simulink model "implementationballandbeam"  (R2015a)
settings: Solver=ode1  StartTime=0.0  StopTime=25  FixedStep=0.002  RelTol=1e-3
libraries: simulink x2, simulink_extras x1
settings Model: ExtModeTrigDuration=5000  Creator=yejingzhou  LastModifiedBy=yejingzhou
settings SolverCC: PositivePriorityOrder=on
settings OptimizationCC: ExpressionDepthLimit=2147483647
settings DebuggingCC: UnderspecifiedInitializationDetection=Classic  MergeDetectMultiDrivingBlocksExec=none  SolverPrmCheckMsg=warning  StateNameClashWarn=warning
settings RTWCC: SystemTargetFile=quarc_win64.tlc  TemplateMakefile=quarc_default_tmf  Description=QUARC Win64 Target
settings STFCustomTargetCC: TargetLibSuffix=.lib  TargetPreCompLibLocation=C:\PROGRA~3\QUARC\lib\2012b\win64\release  GenerateSampleERTMain=off  GeneratePreprocessorConditionals=Disable all  CombineOutputUpdateFcns=on  ERTCustomFileBanners=off  SupportNonInlinedSFcns=on  SupportVariableSizeSignals=off  MATLABClassNameForMDSCustomization=Simulink.SoftwareTarget.GRTCustomization  CPPClassGenCompliant=on  SystemTargetFile=quarc_win64.tlc
settings GRTTargetCC: TargetPreCompLibLocation=C:\PROGRA~3\QUARC\lib\2012b\win64\release  ParMdlRefBuildCompliant=off  CompOptLevelCompliant=off  ConcurrentExecutionCompliant=off  MatFileLogging=off  ExtMode=on  ExtModeMexFile=quarc_comm

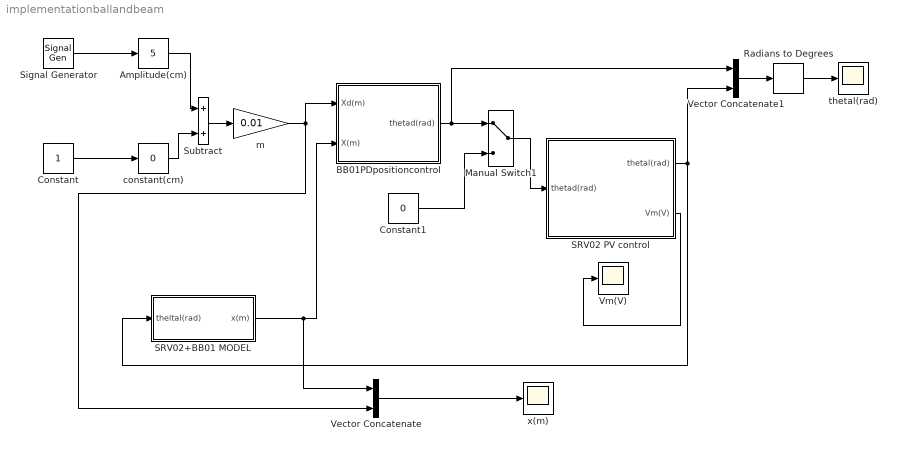
== system implementationballandbeam ==
  Amplitude(cm) : simulink/Math Operations/Slider Gain  low=-1  gain=5  high=10
  BB01PDpositioncontrol : Subsystem
  Constant : Constant
  Constant1 : Constant  Value=0
  Manual Switch1 : ManualSwitch
  Radians to Degrees : simulink_extras/Transformations/Radians to Degrees
  SRV02 PV control : Subsystem
  SRV02+BB01 MODEL : Subsystem
  Signal Generator : SignalGenerator  WaveForm=square  Frequency=0.2  Units=rad/sec
  Subtract : Sum
  Vector Concatenate : Concatenate
  Vector Concatenate1 : Concatenate
  "Vm(V) " : Scope
      settings: SaveName=ScopeData2
  constant(cm) : simulink/Math Operations/Slider Gain  low=0  gain=0  high=5
  "m " : Gain  Gain=0.01
  thetal(rad) : Scope
      settings: TimeRange=25  YMin=-125  YMax=125
  x(m) : Scope
      settings: YMin=-0.09  YMax=0.14
  wires:
  Amplitude(cm)/1 -> Subtract/1
  constant(cm)/1 -> Subtract/2
  Signal Generator/1 -> Amplitude(cm)/1
  Constant/1 -> constant(cm)/1
  Vector Concatenate/1 -> x(m)/1
  Radians to Degrees/1 -> thetal(rad)/1
  BB01PDpositioncontrol/1(thetad(rad)) -> Vector Concatenate1/1, Manual Switch1/1
  Constant1/1 -> Manual Switch1/2
  Manual Switch1/1 -> SRV02 PV control/1(thetad(rad))
  Vector Concatenate1/1 -> Radians to Degrees/1
  SRV02 PV control/1(thetal(rad)) -> SRV02+BB01 MODEL/1(theltal(rad)), Vector Concatenate1/2
  SRV02 PV control/2("Vm(V) ") -> "Vm(V) "/1
  SRV02+BB01 MODEL/1(x(m)) -> Vector Concatenate/1, BB01PDpositioncontrol/2(X(m))
  Subtract/1 -> "m "/1
  "m "/1 -> BB01PDpositioncontrol/1(Xd(m)), Vector Concatenate/2

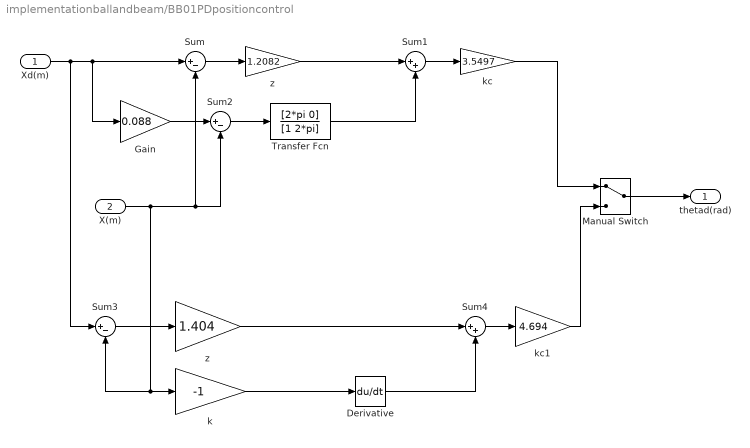
== system implementationballandbeam/BB01PDpositioncontrol ==
  Xd(m) : Inport
  X(m) : Inport  Port=2
  Derivative : Derivative
  Gain : Gain  Gain=0.088
  Manual Switch : ManualSwitch
  Sum : Sum  Inputs=|+-
  Sum1 : Sum  Inputs=|++
  Sum2 : Sum  Inputs=|+-
  Sum3 : Sum  Inputs=|+-
  Sum4 : Sum  Inputs=|++
  Transfer Fcn : TransferFcn  Numerator=[2*pi 0]  Denominator=[1 2*pi]
  k : Gain  Gain=-1
  kc : Gain  Gain=3.5497
  kc1 : Gain  Gain=4.694
  z : Gain  Gain=1.404
  "z " : Gain  Gain=1.2082
  thetad(rad) : Outport
  wires:
  Xd(m)/1 -> Sum/1, Gain/1, Sum3/1
  Sum/1 -> "z "/1
  X(m)/1 -> Sum3/2, k/1, Sum2/2, Sum/2
  "z "/1 -> Sum1/1
  Transfer Fcn/1 -> Sum1/2
  Sum1/1 -> kc/1
  Gain/1 -> Sum2/1
  Sum2/1 -> Transfer Fcn/1
  Sum3/1 -> z/1
  Sum4/1 -> kc1/1
  z/1 -> Sum4/1
  k/1 -> Derivative/1
  Derivative/1 -> Sum4/2
  Manual Switch/1 -> thetad(rad)/1
  kc1/1 -> Manual Switch/2
  kc/1 -> Manual Switch/1

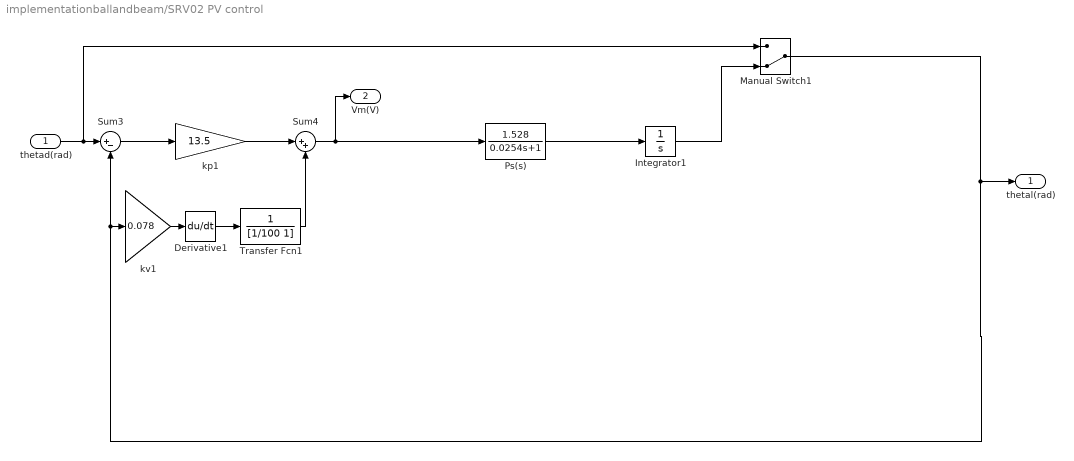
== system implementationballandbeam/SRV02 PV control ==
  thetad(rad) : Inport
  Derivative1 : Derivative
  Integrator1 : Integrator
  Manual Switch1 : ManualSwitch  CurrentSetting=0
  Ps(s) : TransferFcn  Numerator=[1.528]  Denominator=[0.0254 1]
  Sum3 : Sum  Inputs=|+-
  Sum4 : Sum  Inputs=|++
  Transfer Fcn1 : TransferFcn  Denominator=[1/100 1]
  kp1 : Gain  Gain=13.5
  kv1 : Gain  Gain=0.078
  thetal(rad) : Outport
  "Vm(V) " : Outport  Port=2
  wires:
  thetad(rad)/1 -> Manual Switch1/1, Sum3/1
  Sum3/1 -> kp1/1
  kp1/1 -> Sum4/1
  kv1/1 -> Derivative1/1
  Derivative1/1 -> Transfer Fcn1/1
  Transfer Fcn1/1 -> Sum4/2
  Ps(s)/1 -> Integrator1/1
  Manual Switch1/1 -> Sum3/2, kv1/1, thetal(rad)/1
  Sum4/1 -> Ps(s)/1, "Vm(V) "/1
  Integrator1/1 -> Manual Switch1/2

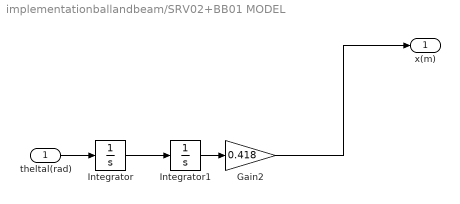
== system implementationballandbeam/SRV02+BB01 MODEL ==
  theltal(rad) : Inport
  Gain2 : Gain  Gain=0.418
  Integrator : Integrator
  Integrator1 : Integrator
  x(m) : Outport
  wires:
  Integrator/1 -> Integrator1/1
  theltal(rad)/1 -> Integrator/1
  Integrator1/1 -> Gain2/1
  Gain2/1 -> x(m)/1
